simulink subsystem "Non_Linear_Model"  (R2024b)
settings: Solver=VariableStepAuto  StartTime=0.0  StopTime=10.0  RelTol=1e-3
settings Model: Creator=alexh  LastModifiedBy=alexh

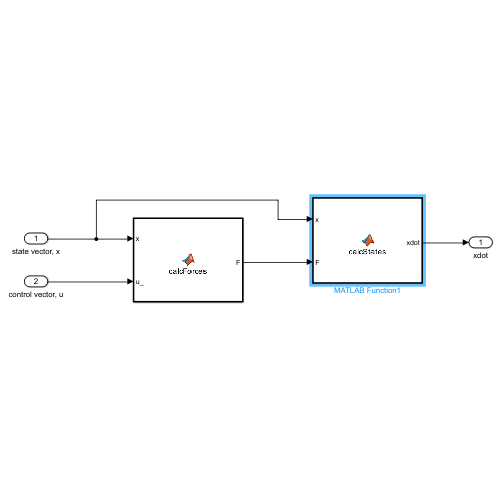
[thumbnail: Simulink's stored preview of the top-level diagram]
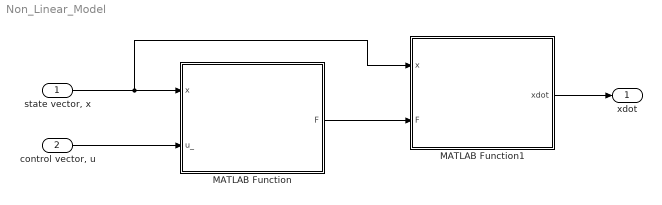
== system Non_Linear_Model ==
  "state vector, x" : Inport
  "control vector, u" : Inport  Port=2
  MATLAB Function : MATLAB Function  TreatAsAtomicUnit=on
  MATLAB Function1 : MATLAB Function  TreatAsAtomicUnit=on
  xdot : Outport
  wires:
  "state vector, x"/1 -> MATLAB Function1/1(x), MATLAB Function/1(x)
  "control vector, u"/1 -> MATLAB Function/2(u_)
  MATLAB Function/1(F) -> MATLAB Function1/2(F)
  MATLAB Function1/1(xdot) -> xdot/1

== matlab function Non_Linear_Model/MATLAB Function1 ==
  data: x input; xdot output; F input
function xdot = calcStates(x,F)

% Extract states
u = x(1);
v = x(2);
w = x(3);
p = x(4);
q = x(5);
r = x(6);
phi = x(7);
theta = x(8);
psi = x(9);

% Extract forces
X = F(1);
Y = F(2);
Z = F(3);
L = F(4);
M = F(5);
N = F(6);

% Calculate xdot
udot = -(m*(q*w - r*v) + g*m*sin(theta) - X)/m;
vdot = (m*(p*w - r*u) + g*m*cos(theta)*sin(phi) + Y)/m;
wdot = (g*m*cos(phi)*cos(theta) - m*(p*v - q*u) + Z)/m;
pdot = (I_xz*(p*q + (p*q*(I_xx - I_yy) - I_xz*q*r + N)/I_zz) + q*r*(I_yy - I_zz) + L)/(- I_xz^2/I_zz + I_xx);
qdot = -(I_xz*(p^2 - r^2) + p*r*(I_xx - I_zz) - M)/I_yy;
rdot = (p*q*(I_xx - I_yy) - I_xz*(q*r - (I_xz*p*q + q*r*(I_yy - I_zz) + L)/I_xx) + N)/(- I_xz^2/I_xx + I_zz);
phidot = p + q*tan(theta)*sin(phi) + r/(tan(theta)*cos(phi)); % NOTE: not valid for for theta=+/-pi/2
thetadot = q*cos(phi) - r*sin(phi);
psidot = q*sin(phi)/cos(theta) + r*cos(phi)/cos(theta); % NOTE: not valid for for theta=+/-pi/2

% Cast into vector
xdot = [udot vdot wdot pdot qdot rdot phidot thetadot psidot];

== matlab function Non_Linear_Model/MATLAB Function ==
  data: x input; u_ input; F output
function F = calcForces(x,u_)

% Extract states
u = x(1);
v = x(2);
w = x(3);
p = x(4);
q = x(5);
r = x(6);
phi = x(7);
theta = x(8);
psi = x(9);

% Extract controls
theta_0 = u_(1);
Delta_theta_0 = u_(2);
theta_1c = u_(3);
theta_1s = u_(4);
delta_r = u_(5);
delta_e = u_(6);

% Calculate forces
